simulink model "cualquiera"  (R2016a)
settings: Solver=VariableStepAuto  StartTime=0.0  StopTime=10.0  RelTol=1e-3
undefined symbols (not defined in the file): pronostico
libraries: fuzblock x1
settings Model: Creator=suare  LastModifiedBy=suare

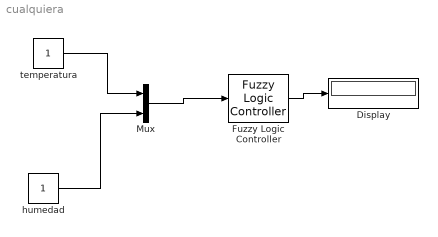
== system cualquiera ==
  Display : Display
  Fuzzy Logic Controller : fuzblock/Fuzzy Logic  Controller  fis=[pronostico]
  Mux : Mux  Inputs=2
  humedad : Constant
  temperatura : Constant
  wires:
  temperatura/1 -> Mux/1
  humedad/1 -> Mux/2
  Mux/1 -> Fuzzy Logic Controller/1
  Fuzzy Logic Controller/1 -> Display/1
